simulink model "final_project"  (R2014a)
settings: Solver=ode45  StartTime=0.0  StopTime=2  RelTol=1e-3
libraries: dsparch4 x3, commnoisgen2 x3, dspsigops x3, commrandsrc2 x1, powerlib_meascontrol x1
settings Model: Creator=pc  LastModifiedBy=pc

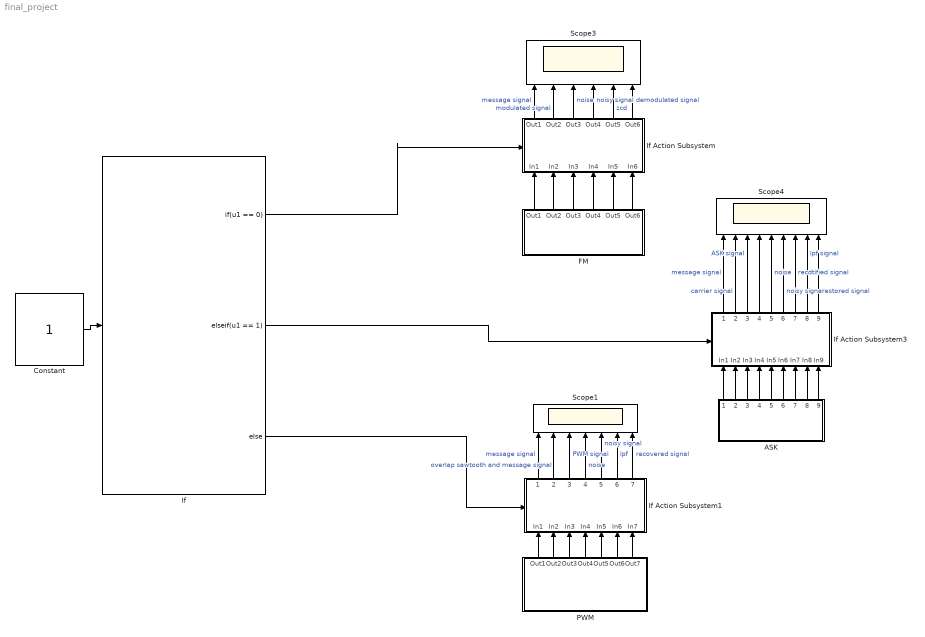
== system final_project ==
  ASK : Subsystem
  Constant : Constant
  FM : Subsystem
  If : If  IfExpression=u1 == 0  ElseIfExpressions=u1 == 1
  If Action Subsystem : Subsystem  TreatAsAtomicUnit=on
  If Action Subsystem1 : Subsystem  TreatAsAtomicUnit=on
  If Action Subsystem3 : Subsystem  TreatAsAtomicUnit=on
  PWM : Subsystem
  Scope1 : Scope  NumInputPorts=7
      settings: YMin=-5~-5~-5~-5~-5~-5~-5  YMax=5~5~5~5~5~5~5
  Scope3 : Scope  NumInputPorts=6
      settings: YMin=-5~-5~-5~-5~-5~-5  YMax=5~5~5~5~5~5
  Scope4 : Scope  NumInputPorts=9
      settings: YMin=-5~-5~-5~-5~-5~-5~-5~-5~-5  YMax=5~5~5~5~5~5~5~5~5  SaveName=ScopeData6
  wires:
  Constant/1 -> If/1
  If/1 -> If Action Subsystem/Action
  ASK/1(Out1) -> If Action Subsystem3/1(In1)
  ASK/2(Out2) -> If Action Subsystem3/2(In2)
  ASK/3(Out3) -> If Action Subsystem3/3(In3)
  ASK/4(Out4) -> If Action Subsystem3/4(In4)
  ASK/6(Out6) -> If Action Subsystem3/6(In6)
  ASK/7(Out7) -> If Action Subsystem3/7(In7)
  ASK/8(Out8) -> If Action Subsystem3/8(In8)
  ASK/9(Out9) -> If Action Subsystem3/9(In9)
  If Action Subsystem3/1(Out1) -> Scope4/1  "message signal"
  If Action Subsystem3/2(Out2) -> Scope4/2  "carrier signal"
  If Action Subsystem3/3(Out3) -> Scope4/3  "ASK signal"
  If Action Subsystem3/4(Out4) -> Scope4/4
  If Action Subsystem3/5(Out5) -> Scope4/5  "noise"
  If Action Subsystem3/6(Out6) -> Scope4/6  "noisy signal"
  If Action Subsystem3/7(Out7) -> Scope4/7  "recdtified signal"
  If Action Subsystem3/8(Out8) -> Scope4/8  "lpf signal"
  If Action Subsystem3/9(Out9) -> Scope4/9  "restored signal"
  If/2 -> If Action Subsystem3/Action
  If/3 -> If Action Subsystem1/Action
  ASK/5(Out5) -> If Action Subsystem3/5(In5)
  PWM/1(Out1) -> If Action Subsystem1/1(In1)
  PWM/2(Out2) -> If Action Subsystem1/2(In2)
  PWM/3(Out3) -> If Action Subsystem1/3(In3)
  PWM/4(Out4) -> If Action Subsystem1/4(In4)
  PWM/5(Out5) -> If Action Subsystem1/5(In5)
  PWM/6(Out6) -> If Action Subsystem1/6(In6)
  PWM/7(Out7) -> If Action Subsystem1/7(In7)
  If Action Subsystem1/1(Out1) -> Scope1/1  "message signal"
  If Action Subsystem1/2(Out2) -> Scope1/2  "overlap sawtooth and message signal"
  If Action Subsystem1/3(Out3) -> Scope1/3  "PWM signal"
  If Action Subsystem1/4(Out4) -> Scope1/4  "noise"
  If Action Subsystem1/5(Out5) -> Scope1/5  "noisy signal"
  If Action Subsystem1/6(Out6) -> Scope1/6  "lpf"
  If Action Subsystem1/7(Out7) -> Scope1/7  "recovered signal"
  FM/1(Out1) -> If Action Subsystem/1(In1)
  FM/2(Out2) -> If Action Subsystem/2(In2)
  FM/3(Out3) -> If Action Subsystem/3(In3)
  FM/4(Out4) -> If Action Subsystem/4(In4)
  FM/5(Out5) -> If Action Subsystem/5(In5)
  FM/6(Out6) -> If Action Subsystem/6(In6)
  If Action Subsystem/1(Out1) -> Scope3/1  "message signal"
  If Action Subsystem/2(Out2) -> Scope3/2  "modulated signal"
  If Action Subsystem/3(Out3) -> Scope3/3  "noise"
  If Action Subsystem/4(Out4) -> Scope3/4  "noisy signal"
  If Action Subsystem/5(Out5) -> Scope3/5  "zcd"
  If Action Subsystem/6(Out6) -> Scope3/6  "demodulated signal"

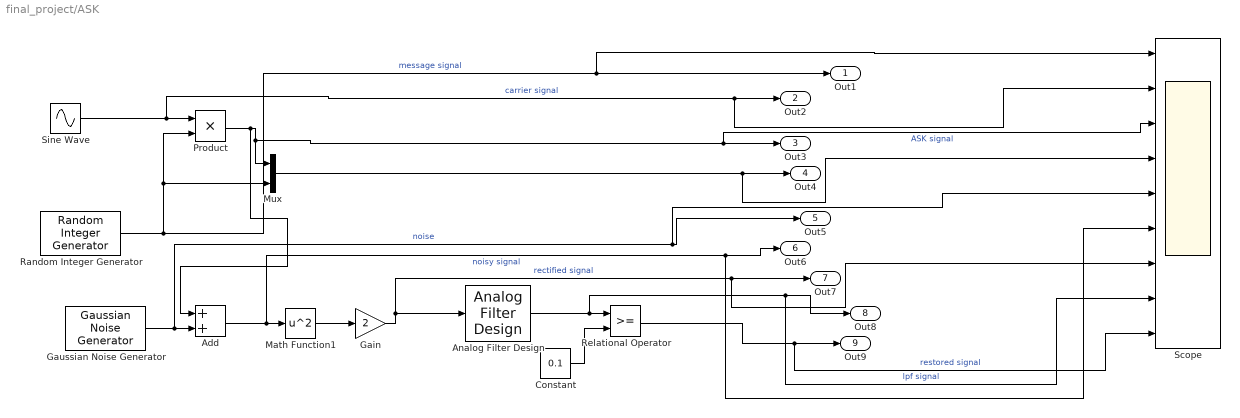
== system final_project/ASK ==
  Add : Sum  SampleTime=.0001
  Analog Filter Design : dsparch4/Analog Filter Design  method=Butterworth  filttype=Lowpass  N=8  Wlo=2*pi*50  Whi=80  Rp=2  Rs=40
  Constant : Constant  Value=0.1  SampleTime=0.0001
  Gain : Gain  Gain=2  SampleTime=0.0001
  Gaussian Noise Generator : commnoisgen2/Gaussian Noise Generator  m=0  d=1e-12  s=41  Ts=0.0001  frameBased=off  sampPerFrame=1  orient=off  outDataType=double
  Math Function1 : Math  Operator=square  SampleTime=.0001  SaturateOnIntegerOverflow=on
  Mux : Mux  Inputs=2
  Product : Product  SampleTime=0.0001
  Random Integer Generator : commrandsrc2/Random Integer Generator  mul=2  seed=37  Ts=.1  frameBased=off  sampPerFrame=1  orient=off  outDataType=double
  Relational Operator : RelationalOperator  OutDataTypeStr=boolean  SampleTime=0.0001
  Scope : Scope  NumInputPorts=9
      settings: YMin=-5~-5~-5~-5~-5~-5~-5~-5~-5  YMax=5~5~5~5~5~5~5~5~5  SaveName=ScopeData3
  Sine Wave : Sin  Frequency=2*pi*50  SampleTime=0.0001
  Out1 : Outport
  Out2 : Outport  Port=2
  Out3 : Outport  Port=3
  Out4 : Outport  Port=4
  Out5 : Outport  Port=5
  Out6 : Outport  Port=6
  Out7 : Outport  Port=7
  Out8 : Outport  Port=8
  Out9 : Outport  Port=9
  wires:
  Sine Wave/1 -> Out2/1, Scope/2, Product/1  "carrier signal"
  Random Integer Generator/1 -> Out1/1, Scope/1, Mux/2, Product/2  "message signal"
  Product/1 -> Add/1, Out3/1, Scope/3, Mux/1  "ASK signal"
  Mux/1 -> Out4/1, Scope/4
  Math Function1/1 -> Gain/1
  Gain/1 -> Out7/1, Scope/7, Analog Filter Design/1  "rectified signal"
  Analog Filter Design/1 -> Out8/1, Scope/8, Relational Operator/1  "lpf signal"
  Constant/1 -> Relational Operator/2
  Gaussian Noise Generator/1 -> Scope/5, Out5/1, Add/2  "noise"
  Add/1 -> Out6/1, Scope/6, Math Function1/1  "noisy signal"
  Relational Operator/1 -> Out9/1, Scope/9  "restored signal"

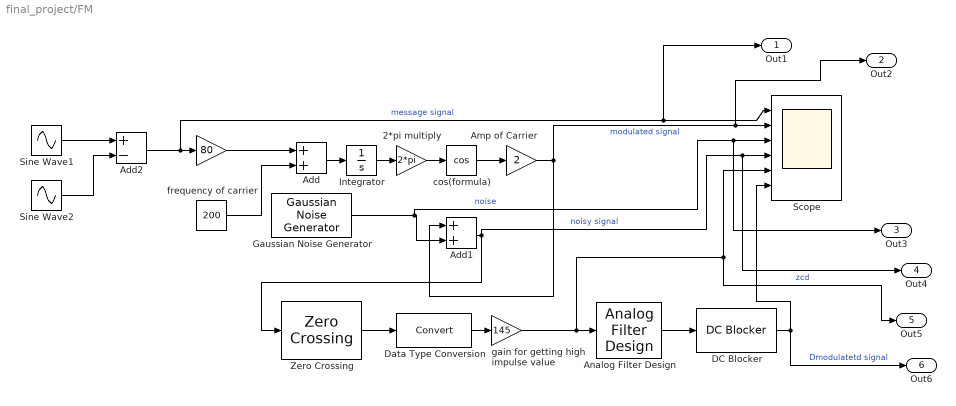
== system final_project/FM ==
  " " : Gain  Gain=80  SampleTime=.0001
  2*pi multiply : Gain  Gain=2*pi  SampleTime=.0001
  Add : Sum  SampleTime=.0001
  Add1 : Sum  SampleTime=.0001
  Add2 : Sum  Inputs=+-  SampleTime=.0001
  Amp of Carrier : Gain  Gain=2  SampleTime=.0001
  Analog Filter Design : dsparch4/Analog Filter Design  method=Butterworth  filttype=Lowpass  N=8  Wlo=2*pi*20  Whi=80  Rp=2  Rs=40
  DC Blocker : dspsigops/DC Blocker  SimulateUsing=Code generation  Algorithm=IIR  NormalizedBandwidth=0.001  Length=8  Order=6
  Data Type Conversion : DataTypeConversion  SampleTime=.0001
  Gaussian Noise Generator : commnoisgen2/Gaussian Noise Generator  m=0  d=0.000001  s=41  Ts=.0001  frameBased=off  sampPerFrame=1  orient=off  outDataType=double
  Integrator : Integrator
  Scope : Scope  NumInputPorts=6
      settings: YMin=-5~-5~-5~-5~-5~-5  YMax=5~5~5~5~5~5  SaveName=ScopeData5
  Sine Wave1 : Sin  Amplitude=4  Frequency=10*pi  SampleTime=.0001
  Sine Wave2 : Sin  Frequency=40*pi  SampleTime=.0001
  Zero Crossing : dspsigops/Zero Crossing  InputProcessing=Columns as channels (frame based)
  cos(formula) : Trigonometry  Operator=cos  SampleTime=.0001
  "frequency of carrier " : Constant  Value=200  SampleTime=.0001
  gain for getting high impulse value : Gain  Gain=145  SampleTime=.0001
  Out1 : Outport
  Out2 : Outport  Port=2
  Out3 : Outport  Port=3
  Out4 : Outport  Port=4
  Out5 : Outport  Port=5
  Out6 : Outport  Port=6
  wires:
  Add2/1 -> " "/1, Out1/1, Scope/1  "message signal"
  " "/1 -> Add/1
  "frequency of carrier "/1 -> Add/2
  Add/1 -> Integrator/1
  Integrator/1 -> 2*pi multiply/1
  2*pi multiply/1 -> cos(formula)/1
  cos(formula)/1 -> Amp of Carrier/1
  Amp of Carrier/1 -> Add1/1, Out2/1, Scope/2  "modulated signal"
  Zero Crossing/1 -> Data Type Conversion/1
  Data Type Conversion/1 -> gain for getting high impulse value/1
  Analog Filter Design/1 -> DC Blocker/1
  Gaussian Noise Generator/1 -> Add1/2, Out3/1, Scope/3  "noise"
  Add1/1 -> Zero Crossing/1, Out4/1, Scope/4  "noisy signal"
  Sine Wave2/1 -> Add2/2
  Sine Wave1/1 -> Add2/1
  DC Blocker/1 -> Scope/6, Out6/1  "Dmodulatetd signal"
  gain for getting high impulse value/1 -> Analog Filter Design/1, Scope/5, Out5/1  "zcd"

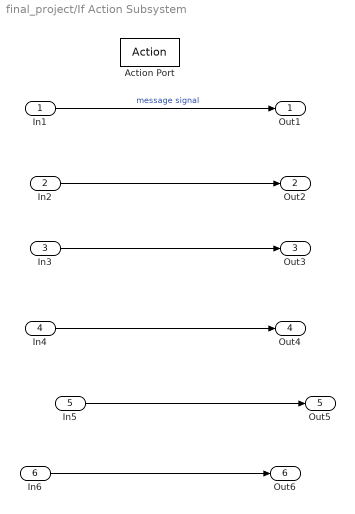
== system final_project/If Action Subsystem ==
  In1 : Inport
  In2 : Inport  Port=2
  In3 : Inport  Port=3
  In4 : Inport  Port=4
  In5 : Inport  Port=5
  In6 : Inport  Port=6
  Action Port : ActionPort  ActionType=then
  Out1 : Outport
  Out2 : Outport  Port=2
  Out3 : Outport  Port=3
  Out4 : Outport  Port=4
  Out5 : Outport  Port=5
  Out6 : Outport  Port=6
  wires:
  In1/1 -> Out1/1  "message signal"
  In2/1 -> Out2/1
  In3/1 -> Out3/1
  In4/1 -> Out4/1
  In5/1 -> Out5/1
  In6/1 -> Out6/1

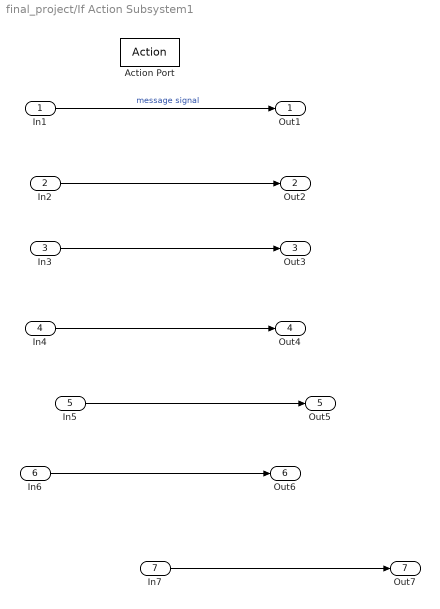
== system final_project/If Action Subsystem1 ==
  In1 : Inport
  In2 : Inport  Port=2
  In3 : Inport  Port=3
  In4 : Inport  Port=4
  In5 : Inport  Port=5
  In6 : Inport  Port=6
  In7 : Inport  Port=7
  Action Port : ActionPort  ActionType=else
  Out1 : Outport
  Out2 : Outport  Port=2
  Out3 : Outport  Port=3
  Out4 : Outport  Port=4
  Out5 : Outport  Port=5
  Out6 : Outport  Port=6
  Out7 : Outport  Port=7
  wires:
  In1/1 -> Out1/1  "message signal"
  In2/1 -> Out2/1
  In3/1 -> Out3/1
  In4/1 -> Out4/1
  In5/1 -> Out5/1
  In6/1 -> Out6/1
  In7/1 -> Out7/1

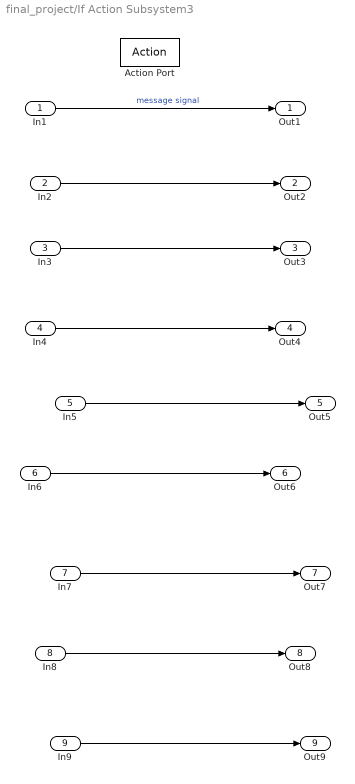
== system final_project/If Action Subsystem3 ==
  In1 : Inport
  In2 : Inport  Port=2
  In3 : Inport  Port=3
  In4 : Inport  Port=4
  In5 : Inport  Port=5
  In6 : Inport  Port=6
  In7 : Inport  Port=7
  In8 : Inport  Port=8
  In9 : Inport  Port=9
  Action Port : ActionPort  ActionType=elseif
  Out1 : Outport
  Out2 : Outport  Port=2
  Out3 : Outport  Port=3
  Out4 : Outport  Port=4
  Out5 : Outport  Port=5
  Out6 : Outport  Port=6
  Out7 : Outport  Port=7
  Out8 : Outport  Port=8
  Out9 : Outport  Port=9
  wires:
  In1/1 -> Out1/1  "message signal"
  In2/1 -> Out2/1
  In3/1 -> Out3/1
  In4/1 -> Out4/1
  In5/1 -> Out5/1
  In6/1 -> Out6/1
  In7/1 -> Out7/1
  In8/1 -> Out8/1
  In9/1 -> Out9/1

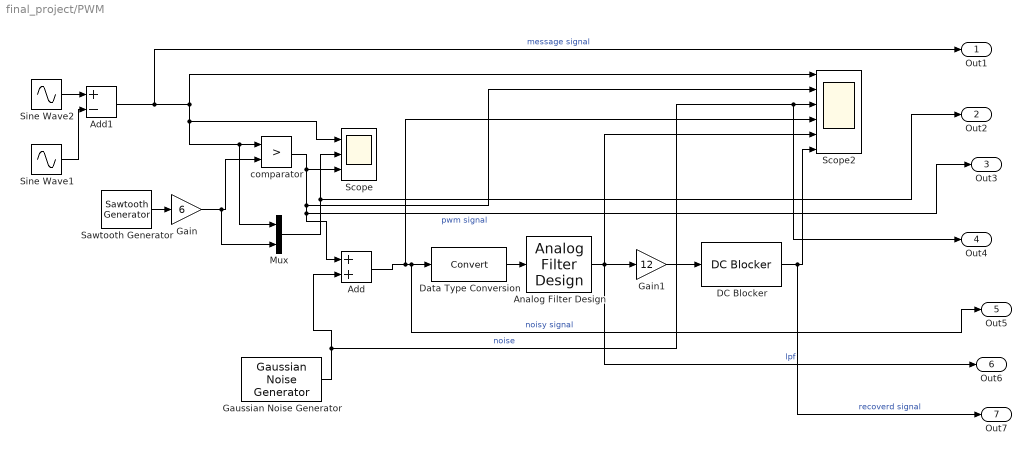
== system final_project/PWM ==
  Add : Sum  SampleTime=0.0001
  Add1 : Sum  Inputs=+-  SampleTime=0.0001
  Analog Filter Design : dsparch4/Analog Filter Design  method=Butterworth  filttype=Lowpass  N=8  Wlo=40*pi  Whi=80  Rp=2  Rs=40
  DC Blocker : dspsigops/DC Blocker  SimulateUsing=Code generation  Algorithm=IIR  NormalizedBandwidth=0.001  Length=8  Order=6
  Data Type Conversion : DataTypeConversion  SampleTime=0.0001
  Gain : Gain  Gain=6  SampleTime=0.0001
  Gain1 : Gain  Gain=12  SampleTime=0.0001
  Gaussian Noise Generator : commnoisgen2/Gaussian Noise Generator  m=0  d=1e-12  s=41  Ts=0.0001  frameBased=off  sampPerFrame=1  orient=off  outDataType=double
  Mux : Mux  Inputs=2
  Sawtooth Generator : powerlib_meascontrol/Pulse & Signal Generators/Sawtooth Generator  Freq=100  Phase=180  Ts=0
  Scope : Scope  NumInputPorts=3
      settings: YMin=-5~-5~-5  YMax=5~5~5  SaveName=ScopeData4
  Scope2 : Scope  NumInputPorts=6
      settings: YMin=-5~-5~-5~-5~-5~-5  YMax=5~5~5~5~5~5  SaveName=ScopeData2
  Sine Wave1 : Sin  Amplitude=4  Frequency=10*pi  SampleTime=0.0001
  Sine Wave2 : Sin  Frequency=40*pi  SampleTime=0.0001
  "comparator " : RelationalOperator  Operator=>  OutDataTypeStr=boolean  SampleTime=0.0001
  Out1 : Outport
  Out2 : Outport  Port=2
  Out3 : Outport  Port=3
  Out4 : Outport  Port=4
  Out5 : Outport  Port=5
  Out6 : Outport  Port=6
  Out7 : Outport  Port=7
  wires:
  Mux/1 -> Scope/2, Out2/1
  "comparator "/1 -> Out3/1, Add/1, Scope2/2, Scope/3  "pwm signal"
  Gain/1 -> Mux/2, "comparator "/2
  Sawtooth Generator/1 -> Gain/1
  Data Type Conversion/1 -> Analog Filter Design/1
  Analog Filter Design/1 -> Out6/1, Gain1/1, Scope2/5  "lpf"
  Gaussian Noise Generator/1 -> Add/2, Out4/1, Scope2/3  "noise"
  Add/1 -> Out5/1, Data Type Conversion/1, Scope2/4  "noisy signal"
  DC Blocker/1 -> Out7/1, Scope2/6  "recoverd signal"
  Gain1/1 -> DC Blocker/1
  Sine Wave1/1 -> Add1/2
  Sine Wave2/1 -> Add1/1
  Add1/1 -> Out1/1, Scope/1, Mux/1, "comparator "/1, Scope2/1  "message signal"
